simulink model "bnew"  (Simulink 7.4)
settings: Solver=FixedStepDiscrete  StartTime=0.0  StopTime=0.25  FixedStep=Ts  RelTol=1e-3
values from neighbouring files (symbols this model uses):
  Ts = 1/fs    (= 1e-05)    [RunBearing1.m]
undefined symbols (not defined in the file or in its folder): DiscIntNeverNeededParam
libraries: powerlib x1
settings Model: Creator=rohank  LastModifiedBy=rohank
settings CodeAppCC: CustomSymbolStrType=$N$R$M_T
settings SimEventsCC: propDiagAttribOutput=1  propDiagFcnCallOutput=1  propDiagStatOutput=0

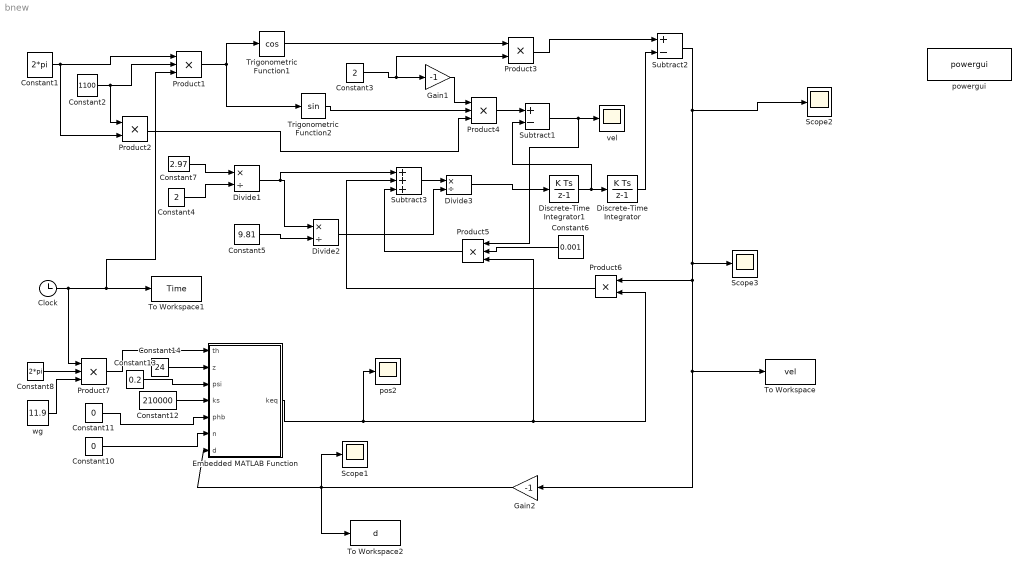
== system bnew ==
  Clock : Clock
      settings: Decimation=10
  Constant1 : Constant  Value=2*pi
  Constant10 : Constant  Value=0
  Constant11 : Constant  Value=0
  Constant12 : Constant  Value=210000
  Constant13 : Constant  Value=0.2
  Constant14 : Constant  Value=24
  Constant2 : Constant  Value=1100
  Constant3 : Constant  Value=2
  Constant4 : Constant  Value=2
  Constant5 : Constant  Value=9.81
  Constant6 : Constant  Value=0.001
  Constant7 : Constant  Value=2.97
  Constant8 : Constant  Value=2*pi
  Discrete-Time Integrator : DiscreteIntegrator  SampleTime=Ts  ICPrevOutput=DiscIntNeverNeededParam  ICPrevScaledInput=DiscIntNeverNeededParam
  Discrete-Time Integrator1 : DiscreteIntegrator  SampleTime=Ts  ICPrevOutput=DiscIntNeverNeededParam  ICPrevScaledInput=DiscIntNeverNeededParam
  Divide1 : Product  Inputs=*/
  Divide2 : Product  Inputs=*/
  Divide3 : Product  Inputs=*/
  Embedded MATLAB Function : Subsystem  TreatAsAtomicUnit=on
  Gain1 : Gain  Gain=-1
  Gain2 : Gain  Gain=-1
  Product{1,4..5,7} (4 alike) : Product  Inputs=3  RndMeth=Zero
  Product2 : Product  RndMeth=Zero
  Product3 : Product  RndMeth=Zero
  Product6 : Product  RndMeth=Zero
  Scope1 : Scope
      settings: SaveName=vib
  Scope2 : Scope
      settings: TimeRange=0.25  YMin=-3  YMax=4  SaveName=sc  DataFormat=Array
  Scope3 : Scope
      settings: SaveName=vib2
  Subtract1 : Sum  Inputs=+-
  Subtract2 : Sum  Inputs=+-
  Subtract3 : Sum  Inputs=+++
  To Workspace : ToWorkspace  VariableName=vel  SampleTime=-1  SaveFormat=Structure
  To Workspace1 : ToWorkspace  VariableName=Time  SampleTime=-1  SaveFormat=Structure
  To Workspace2 : ToWorkspace  VariableName=d  SampleTime=-1  SaveFormat=Array
  Trigonometric Function1 : Trigonometry  Operator=cos
  Trigonometric Function2 : Trigonometry
  pos2 : Scope
      settings: TimeRange=0.5999999999999996  YMin=1625128  YMax=1625130.5  SaveName=ScopeData4
  powergui : powerlib/powergui  Priority=1  SystemSampleTime=-1  SimulationMode=Discrete  SampleTime=Ts  frequency=60  SPID=off  DisableSnubberDevices=off  DisableRonSwitches=off  DisableVfSwitches=off  SwTol=0  Interpol=off  frequencyindice=60  echomessages=off  HookPort=off  DisplayEquations=off  FunctionMessages=off  EnableUseOfTLC=off  x0status=blocks  RestoreLinks=warning  Frange=[0:2:500]  Ylog=off  Xlog=on  ShowGrid=off  save=off  variable=ZData  structure=vib  ZoomFFT=off  StartTime=0.03  cycles=15  DisplayStyle=1  fundamental=11.9  FreqAxis=off  MaxFrequency=200  frequencyindicesteady=1  RmsSteady=1  display=off  Ts=0  methode=off
  vel : Scope
      settings: SaveName=vib3
  wg : Constant  Value=11.9
  wires:
  Constant1/1 -> Product1/1, Product2/2
  Constant2/1 -> Product1/2, Product2/1
  Product1/1 -> Trigonometric Function1/1, Trigonometric Function2/1
  Trigonometric Function1/1 -> Product3/1
  Constant3/1 -> Gain1/1, Product3/2
  Gain1/1 -> Product4/1
  Trigonometric Function2/1 -> Product4/2
  Product2/1 -> Product4/3
  Product4/1 -> Subtract1/1
  Subtract1/1 -> Product5/1, vel/1
  Product3/1 -> Subtract2/1
  Constant7/1 -> Divide1/1
  Constant4/1 -> Divide1/2
  Divide1/1 -> Divide2/1, Subtract3/1
  Constant5/1 -> Divide2/2
  Subtract3/1 -> Divide3/1
  Divide2/1 -> Divide3/2
  Divide3/1 -> Discrete-Time Integrator1/1
  Discrete-Time Integrator1/1 -> Subtract1/2, Discrete-Time Integrator/1
  Discrete-Time Integrator/1 -> Subtract2/2
  Product5/1 -> Subtract3/3
  Constant6/1 -> Product5/2
  Product6/1 -> Subtract3/2
  Subtract2/1 -> To Workspace/1, Gain2/1, Product6/1, Scope3/1, Scope2/1
  Embedded MATLAB Function/1(keq) -> Product6/2, Product5/3, pos2/1
  Clock/1 -> To Workspace1/1, Product1/3, Product7/1
  wg/1 -> Product7/3
  Constant8/1 -> Product7/2
  Constant10/1 -> Embedded MATLAB Function/6(n)
  Constant11/1 -> Embedded MATLAB Function/5(phb)
  Constant12/1 -> Embedded MATLAB Function/4(ks)
  Constant13/1 -> Embedded MATLAB Function/3(psi)
  Constant14/1 -> Embedded MATLAB Function/2(z)
  Product7/1 -> Embedded MATLAB Function/1(th)
  Gain2/1 -> To Workspace2/1, Scope1/1, Embedded MATLAB Function/7(d)

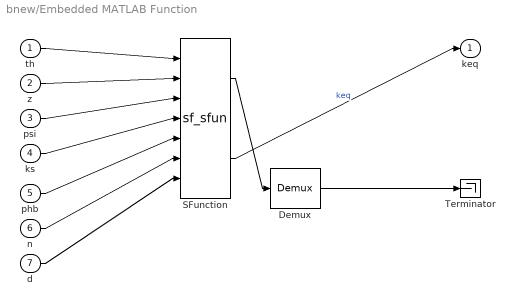
== system bnew/Embedded MATLAB Function ==
  th : Inport
  z : Inport  Port=2
  psi : Inport  Port=3
  ks : Inport  Port=4
  phb : Inport  Port=5
  n : Inport  Port=6
  d : Inport  Port=7
  " Demux " : Demux  Outputs=1
  " SFunction " : S-Function  Tag=Stateflow S-Function bnew 2  FunctionName=sf_sfun  PortCounts=[7 2]  EnableBusSupport=on
  " Terminator " : Terminator
  keq : Outport
  wires:
  th/1 -> " SFunction "/1
  z/1 -> " SFunction "/2
  psi/1 -> " SFunction "/3
  ks/1 -> " SFunction "/4
  phb/1 -> " SFunction "/5
  n/1 -> " SFunction "/6
  d/1 -> " SFunction "/7
  " SFunction "/2 -> keq/1  "keq"
  " Demux "/1 -> " Terminator "/1
  " SFunction "/1 -> " Demux "/1

== matlab function Embedded MATLAB Function ==
  data: th input double; keq output double; z input double; psi input double; ks input double; phb input double; n input double; d input double
function keq = fcn(th,z,psi,ks,phb,n,d )
%#eml

% hole=(2*pi/z)*(n+1);
% th_i=theta_g+ph_b;
% th_f=theta_g+ph_b+hole;
% keq=0;
% for i=1:z
%     Theta=theta_g+((2*pi)/z)*(i-1)+psi-pi;
%     delta=cos(Theta);
%     if (sign(delta)>=0) && ((Theta<th_i) || (Theta>th_f)) && (d<0)
%         keq=keq+delta*ks;
%     elseif (sign(delta)<0) && ((Theta<th_i) || (Theta>th_f)) && (d>=0)
%         keq=keq-delta*ks;
%     end
% end


y=0;
a=0;
j=1;
sum=0;
k=1;
v=0;
for j=1:24
    v=( (j*2*pi)/z );
    if (v>=0  && v<=(  ((n)*2*pi)/z)  )
        k=0;
    else
        k=1;
    end
    b= (sign(psi + d));
    x= sign(  cos( ( th + (j*2*pi)/z ) ) );
    
    if b==0 || x==0
        h=0;
    
    elseif b==x
        h=1;
    
    else
        h=0;
    end
    
    
    y= cos( ( th + (j*2*pi)/z) );
    a=abs( power(complex(y),2.5));
    sum= sum + (a*k*h); 
    
end

keq= ks*sum;
